simulink model "modelo_linear_v2"  (R2014b)
settings: Solver=ode45  StartTime=0.0  StopTime=T_sim  RelTol=1e-3
InitFcn:
  | main_v2
values from neighbouring files (symbols this model uses):
  Aw = A22(1:3,1:3)    [main_model2.m]    (also in main_modelo_linear_v1.m; main_modelo_linear_v2.m = zeros(6,6); main_modelo_nao_linear_v2.m)
  Bw = B22(1:3,1:3)    [main_model2.m]    (also in main_modelo_linear_v1.m; main_modelo_linear_v2.m = zeros(6,3); main_modelo_nao_linear_v2.m)
  Cw = eye(3)    [main_model2.m]    (also in main_modelo_linear_v1.m; main_modelo_linear_v2.m = eye(6); main_modelo_nao_linear_v2.m)
  Dw = zeros(3)    [main_model2.m]    (also in main_modelo_linear_v1.m; main_modelo_linear_v2.m = zeros(6,3); main_modelo_nao_linear_v2.m)
  g = 9.8    [main_model1.m]    (also in main_model2.m; main_modelo_linear_v1.m; main_modelo_linear_v2.m; main_modelo_nao_linear_v1.m)
  Kd_rot = 0.01    [main_model1.m]    (also in main_model2.m; main_modelo_linear_v1.m = 0; main_modelo_linear_v2.m = 0; main_modelo_nao_linear_v1.m)
  Kd_trans = 0.002    [main_model1.m]    (also in main_model2.m = -0.13723; main_modelo_linear_v1.m = 0; main_modelo_linear_v2.m = 0; main_modelo_nao_linear_v1.m)
  Ki_rot = 1.0    (= 1)    [main_model1.m]    (also in main_model2.m; main_modelo_linear_v1.m = 0.5; main_modelo_linear_v2.m = 0.5; main_modelo_nao_linear_v1.m)
  Ki_trans = 0.06    [main_model1.m]    (also in main_model2.m = 0.41774; main_modelo_linear_v1.m = 0; main_modelo_linear_v2.m = 1; main_modelo_nao_linear_v1.m)
  Kp_rot = 10    [main_model1.m]    (also in main_model2.m; main_modelo_linear_v1.m = 1; main_modelo_linear_v2.m = 1; main_modelo_nao_linear_v1.m)
  Kp_trans = 0.4    [main_model1.m]    (also in main_model2.m = 2.0968; main_modelo_linear_v1.m = 1; main_modelo_linear_v2.m = 2; main_modelo_nao_linear_v1.m)
  m = 1.0428    [main_model1.m]    (also in main_model2.m; main_modelo_linear_v1.m = 1; main_modelo_linear_v2.m = 1; main_modelo_nao_linear_v1.m)
  p0 = 0    [main_model2.m]    (also in main_modelo_linear_v1.m; main_modelo_linear_v2.m; main_modelo_nao_linear_v2.m; modelo_naolinear.m)
  phi0 = 0    [main_model1.m]    (also in main_model2.m; main_modelo_linear_v1.m; main_modelo_linear_v2.m; main_modelo_nao_linear_v1.m)
  psi0 = 0    [main_model1.m]    (also in main_model2.m; main_modelo_linear_v1.m; main_modelo_linear_v2.m; main_modelo_nao_linear_v1.m)
  q0 = 0    [main_model2.m]    (also in main_modelo_linear_v1.m; main_modelo_linear_v2.m; main_modelo_nao_linear_v2.m; modelo_naolinear.m)
  r0 = 0    [main_model2.m]    (also in main_modelo_linear_v1.m; main_modelo_linear_v2.m; main_modelo_nao_linear_v2.m; modelo_naolinear.m)
  theta0 = 0    [main_model1.m]    (also in main_model2.m; main_modelo_linear_v1.m; main_modelo_linear_v2.m; main_modelo_nao_linear_v1.m)
  vxd = 0    [main_model1.m]    (also in main_model2.m; main_modelo_linear_v1.m; main_modelo_linear_v2.m; main_modelo_nao_linear_v1.m)
  vyd = 0    [main_model1.m]    (also in main_model2.m; main_modelo_linear_v1.m; main_modelo_linear_v2.m; main_modelo_nao_linear_v1.m)
  x0 = 0    [main_model1.m]    (also in main_model2.m; main_modelo_linear_v1.m; main_modelo_linear_v2.m; main_modelo_nao_linear_v1.m)
  y0 = 0    [main_model1.m]    (also in main_model2.m; main_modelo_linear_v1.m; main_modelo_linear_v2.m; main_modelo_nao_linear_v1.m)
  z0 = 1    [main_model1.m]    (also in main_model2.m; main_modelo_linear_v1.m; main_modelo_linear_v2.m; main_modelo_nao_linear_v1.m)
undefined symbols (not defined in the file or in its folder): sigbuilder_block
libraries: simulink x6
settings Model: Creator=dferr  LastModifiedBy=dferr
settings DebuggingCC: SolverPrmCheckMsg=none

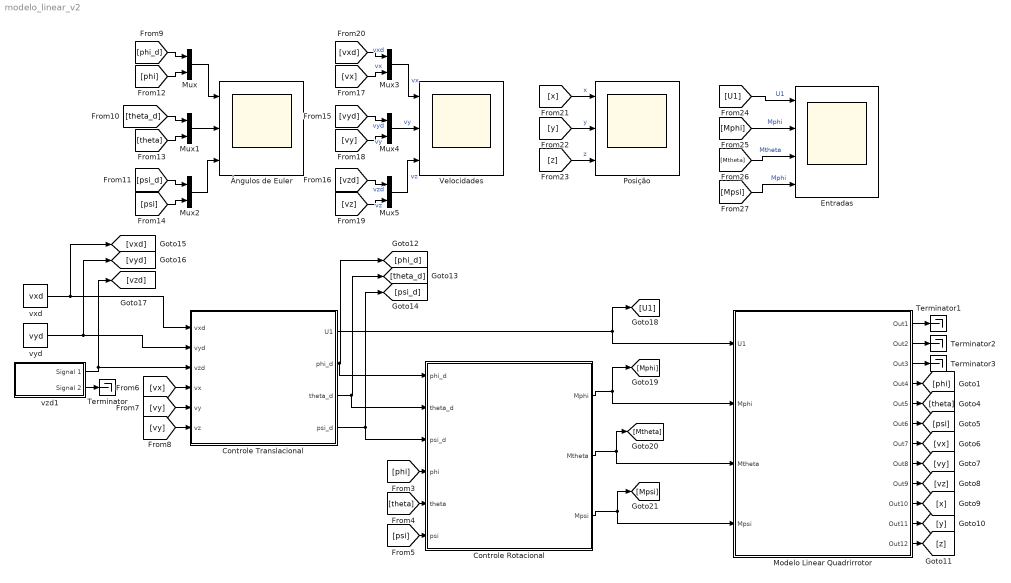
== system modelo_linear_v2 ==
  Controle Rotacional : Subsystem
      mask Display:
      | disp('Controle Rotacional')
      | port_label('input',1,'phi_d')
      | port_label('input',2,'theta_d')
      | port_label('input',3,'psi_d')
      | port_label('input',4,'phi')
      | port_label('input',5,'theta')
      | port_label('input',6,'psi')
      | port_label('output',1,'Mphi')
      | port_label('output',2,'Mtheta')
      | port_label('output',3,'Mpsi')
  Controle Translacional : Subsystem
      mask Display:
      | disp('Controle Translacional')
      | port_label('input',1,'vxd')
      | port_label('input',2,'vyd')
      | port_label('input',3,'vzd')
      | port_label('input',4,'vx')
      | port_label('input',5,'vy')
      | port_label('input',6,'vz')
      | port_label('output',1,'U1')
      | port_label('output',2,'phi_d')
      | port_label('output',3,'theta_d')
      | port_label('output',4,'psi_d')
  Entradas : Scope  NumInputPorts=4
      settings: YMin=-5~-5~-5~-5  YMax=5~5~5~5  SaveName=ScopeData3
  Modelo Linear Quadrirrotor : Subsystem
      mask Display:
      | disp('Modelo Linear Quadrirrotor')
      | port_label('input',1,'U1')
      | port_label('input',2,'Mphi')
      | port_label('input',3,'Mtheta')
      | port_label('input',4,'Mpsi')
      | port_label('output',1,'p')
      | port_label('output',2,'q')
      | port_label('output',3,'r')
      | port_label('output',4,'phi')
      | port_label('output',5,'theta')
      | port_label('output',6,'psi')
      | port_label('output',7,'vx')
      | port_label('output',8,'vy')
      | port_label('output',9,'vz')
      | port_label('output',10,'x')
      | port_label('output',11,'y')
      | port_label('output',12,'z')
  Mux{,1..5} (6 alike) : Mux  Inputs=2
  Posição : Scope  NumInputPorts=3
      settings: YMin=-5~-5~-5  YMax=5~5~5  SaveName=ScopeData2
  Terminator{,1..3} (4 alike) : Terminator
  Velocidades : Scope  NumInputPorts=3
      settings: ShowLegends=on  YMin=-5~-5~-5  YMax=5~5~5
  vxd : Constant  Value=vxd
  vyd : Constant  Value=vyd
  vzd1 : Subsystem  Tag=STV Subsys  LoadFcn=sigbuilder_block('load');  StartFcn=sigbuilder_block('start');  StopFcn=sigbuilder_block('stop');  ClipboardFcn=sigbuilder_block('clipboard');  mask(Sigbuilder block){}
      mask help: Simulink:masks:SigbuilderBlock_MD
      mask init:
      | if ~strcmp(get_param(bdroot(gcbh),'SimulationStatus'),'stopped') tuvar = sigbuilder_block('maskInit'); end
      settings: CopyFcn=sigbuilder_block('copy');  DeleteFcn=sigbuilder_block('delete');  ModelCloseFcn=sigbuilder_block('modelClose');  PreSaveFcn=sigbuilder_block('preSave');  PauseFcn=sigbuilder_block('pause');  ContinueFcn=sigbuilder_block('continue');  NameChangeFcn=sigbuilder_block('namechange');  OpenFcn=sigbuilder_block('open',[437.6 199.2 550.4 400 ]);  CloseFcn=sigbuilder_block('close');
      mask Display: plot(0, 0, 100, 100,[2, 2, 32, 32, 2], [68, 8, 8, 68, 68],[32, 2], [38, 38], [32, 19, 2],[53, 60, 44], [32, 17, 17, 2],[16, 16, 31, 31]);txt = getActiveGroup(gcbh);text(2, 100, txt,'verticalAlignment', 'top');
  Ângulos de Euler : Scope  NumInputPorts=3
      settings: YMin=-5~-5~-5  YMax=5~5~5
  wires:
  Controle Rotacional/1(Mphi) -> [Mphi], Modelo Linear Quadrirrotor/2(Mphi)
  Controle Rotacional/2(Mtheta) -> [Mtheta], Modelo Linear Quadrirrotor/3(Mtheta)
  Controle Rotacional/3(Mpsi) -> [Mpsi], Modelo Linear Quadrirrotor/4(Mpsi)
  Controle Translacional/4(psi_d) -> [psi_d], Controle Rotacional/3(psi_d)
  Controle Translacional/3(theta_d) -> Controle Rotacional/2(theta_d), [theta_d]
  Controle Translacional/2(phi_d) -> Controle Rotacional/1(phi_d), [phi_d]
  Controle Translacional/1(U1) -> [U1], Modelo Linear Quadrirrotor/1(U1)
  [vx] -> Controle Translacional/4(vx)
  [vy] -> Controle Translacional/5(vy)
  [vy] -> Controle Translacional/6(vz)
  vyd/1 -> [vyd], Controle Translacional/2(vyd)
  vxd/1 -> [vxd], Controle Translacional/1(vxd)
  [phi] -> Mux/2
  [phi_d] -> Mux/1
  [theta_d] -> Mux1/1
  [theta] -> Mux1/2
  [psi_d] -> Mux2/1
  [psi] -> Mux2/2
  Mux1/1 -> Ângulos de Euler/2
  Mux/1 -> Ângulos de Euler/1
  Mux2/1 -> Ângulos de Euler/3
  vzd1/2(Signal 2) -> Terminator/1
  [vx] -> Mux3/2  "vx"
  [vxd] -> Mux3/1  "vxd"
  [vyd] -> Mux4/1  "vyd"
  [vy] -> Mux4/2  "vy"
  [vzd] -> Mux5/1  "vzd"
  [vz] -> Mux5/2  "vz"
  Mux4/1 -> Velocidades/2  "vy"
  Mux3/1 -> Velocidades/1  "vx"
  Mux5/1 -> Velocidades/3  "vz"
  [x] -> Posição/1  "x"
  [y] -> Posição/2  "y"
  [z] -> Posição/3  "z"
  [U1] -> Entradas/1  "U1"
  [Mphi] -> Entradas/2  "Mphi"
  [Mtheta] -> Entradas/3  "Mtheta"
  [Mpsi] -> Entradas/4  "Mphi"
  vzd1/1(Signal 1) -> Controle Translacional/3(vzd), [vzd]
  Modelo Linear Quadrirrotor/1(Out1) -> Terminator1/1
  Modelo Linear Quadrirrotor/2(Out2) -> Terminator2/1
  Modelo Linear Quadrirrotor/3(Out3) -> Terminator3/1
  Modelo Linear Quadrirrotor/4(Out4) -> [phi]
  Modelo Linear Quadrirrotor/5(Out5) -> [theta]
  Modelo Linear Quadrirrotor/6(Out6) -> [psi]
  Modelo Linear Quadrirrotor/7(Out7) -> [vx]
  Modelo Linear Quadrirrotor/8(Out8) -> [vy]
  Modelo Linear Quadrirrotor/9(Out9) -> [vz]
  Modelo Linear Quadrirrotor/10(Out10) -> [x]
  Modelo Linear Quadrirrotor/11(Out11) -> [y]
  Modelo Linear Quadrirrotor/12(Out12) -> [z]
  [phi] -> Controle Rotacional/4(phi)
  [theta] -> Controle Rotacional/5(theta)
  [psi] -> Controle Rotacional/6(psi)

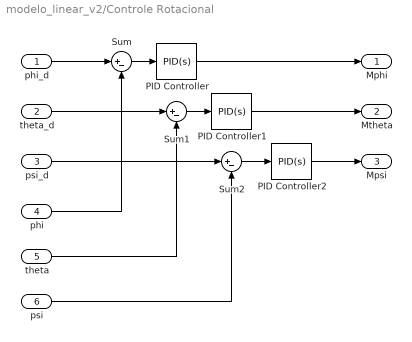
== system modelo_linear_v2/Controle Rotacional ==
  phi_d : Inport
  theta_d : Inport  Port=2
  psi_d : Inport  Port=3
  phi : Inport  Port=4
  theta : Inport  Port=5
  psi : Inport  Port=6
  PID Controller : simulink/Continuous/PID Controller  Controller=PID  TimeDomain=Continuous-time  SampleTime=-1  IntegratorMethod=Forward Euler  FilterMethod=Forward Euler  Form=Parallel  P=Kp_rot  I=Ki_rot  D=Kd_rot  N=100  InitialConditionSource=internal  InitialConditionForIntegrator=0  InitialConditionForFilter=0  ExternalReset=none  LimitOutput=off  UpperSaturationLimit=inf  LowerSaturationLimit=-inf  LinearizeAsGain=on  AntiWindupMode=none  Kb=1  TrackingMode=off  Kt=1  PParamMin=[]  PParamMax=[]  IParamMin=[]  IParamMax=[]  DParamMin=[]  DParamMax=[]  NParamMin=[]  NParamMax=[]  KbParamMin=[]  KbParamMax=[]  KtParamMin=[]  KtParamMax=[]  POutMin=[]  POutMax=[]  IOutMin=[]  IOutMax=[]  DOutMin=[]  DOutMax=[]  NOutMin=[]  NOutMax=[]  KbOutMin=[]  KbOutMax=[]  KtOutMin=[]  KtOutMax=[]  IntegratorOutMin=[]  IntegratorOutMax=[]  FilterOutMin=[]  FilterOutMax=[]  SumOutMin=[]  SumOutMax=[]  SumI1OutMin=[]  SumI1OutMax=[]  SumI2OutMin=[]  SumI2OutMax=[]  SumI3OutMin=[]  SumI3OutMax=[]  SumDOutMin=[]  SumDOutMax=[]  SaturationOutMin=[]  SaturationOutMax=[]  IntegratorContinuousStateAttributes=''  IntegratorStateMustResolveToSignalObject=off  IntegratorRTWStateStorageClass=Auto  FilterContinuousStateAttributes=''  FilterStateMustResolveToSignalObject=off  FilterRTWStateStorageClass=Auto  DifferentiatorICPrevScaledInput=0  DifferentiatorOutMin=[]  DifferentiatorOutMax=[]  UseFilter=on
  PID Controller1 : simulink/Continuous/PID Controller  Controller=PID  TimeDomain=Continuous-time  SampleTime=-1  IntegratorMethod=Forward Euler  FilterMethod=Forward Euler  Form=Parallel  P=Kp_rot  I=Ki_rot  D=Kd_rot  N=100  InitialConditionSource=internal  InitialConditionForIntegrator=0  InitialConditionForFilter=0  ExternalReset=none  LimitOutput=off  UpperSaturationLimit=inf  LowerSaturationLimit=-inf  LinearizeAsGain=on  AntiWindupMode=none  Kb=1  TrackingMode=off  Kt=1  PParamMin=[]  PParamMax=[]  IParamMin=[]  IParamMax=[]  DParamMin=[]  DParamMax=[]  NParamMin=[]  NParamMax=[]  KbParamMin=[]  KbParamMax=[]  KtParamMin=[]  KtParamMax=[]  POutMin=[]  POutMax=[]  IOutMin=[]  IOutMax=[]  DOutMin=[]  DOutMax=[]  NOutMin=[]  NOutMax=[]  KbOutMin=[]  KbOutMax=[]  KtOutMin=[]  KtOutMax=[]  IntegratorOutMin=[]  IntegratorOutMax=[]  FilterOutMin=[]  FilterOutMax=[]  SumOutMin=[]  SumOutMax=[]  SumI1OutMin=[]  SumI1OutMax=[]  SumI2OutMin=[]  SumI2OutMax=[]  SumI3OutMin=[]  SumI3OutMax=[]  SumDOutMin=[]  SumDOutMax=[]  SaturationOutMin=[]  SaturationOutMax=[]  IntegratorContinuousStateAttributes=''  IntegratorStateMustResolveToSignalObject=off  IntegratorRTWStateStorageClass=Auto  FilterContinuousStateAttributes=''  FilterStateMustResolveToSignalObject=off  FilterRTWStateStorageClass=Auto  DifferentiatorICPrevScaledInput=0  DifferentiatorOutMin=[]  DifferentiatorOutMax=[]  UseFilter=on
  PID Controller2 : simulink/Continuous/PID Controller  Controller=PID  TimeDomain=Continuous-time  SampleTime=-1  IntegratorMethod=Forward Euler  FilterMethod=Forward Euler  Form=Parallel  P=Kp_rot  I=Ki_rot  D=Kd_rot  N=100  InitialConditionSource=internal  InitialConditionForIntegrator=0  InitialConditionForFilter=0  ExternalReset=none  LimitOutput=off  UpperSaturationLimit=inf  LowerSaturationLimit=-inf  LinearizeAsGain=on  AntiWindupMode=none  Kb=1  TrackingMode=off  Kt=1  PParamMin=[]  PParamMax=[]  IParamMin=[]  IParamMax=[]  DParamMin=[]  DParamMax=[]  NParamMin=[]  NParamMax=[]  KbParamMin=[]  KbParamMax=[]  KtParamMin=[]  KtParamMax=[]  POutMin=[]  POutMax=[]  IOutMin=[]  IOutMax=[]  DOutMin=[]  DOutMax=[]  NOutMin=[]  NOutMax=[]  KbOutMin=[]  KbOutMax=[]  KtOutMin=[]  KtOutMax=[]  IntegratorOutMin=[]  IntegratorOutMax=[]  FilterOutMin=[]  FilterOutMax=[]  SumOutMin=[]  SumOutMax=[]  SumI1OutMin=[]  SumI1OutMax=[]  SumI2OutMin=[]  SumI2OutMax=[]  SumI3OutMin=[]  SumI3OutMax=[]  SumDOutMin=[]  SumDOutMax=[]  SaturationOutMin=[]  SaturationOutMax=[]  IntegratorContinuousStateAttributes=''  IntegratorStateMustResolveToSignalObject=off  IntegratorRTWStateStorageClass=Auto  FilterContinuousStateAttributes=''  FilterStateMustResolveToSignalObject=off  FilterRTWStateStorageClass=Auto  DifferentiatorICPrevScaledInput=0  DifferentiatorOutMin=[]  DifferentiatorOutMax=[]  UseFilter=on
  Sum : Sum  Inputs=|+-
  Sum1 : Sum  Inputs=|+-
  Sum2 : Sum  Inputs=|+-
  Mphi : Outport
  Mtheta : Outport  Port=2
  Mpsi : Outport  Port=3
  wires:
  PID Controller1/1 -> Mtheta/1
  PID Controller/1 -> Mphi/1
  PID Controller2/1 -> Mpsi/1
  Sum/1 -> PID Controller/1
  Sum1/1 -> PID Controller1/1
  Sum2/1 -> PID Controller2/1
  phi_d/1 -> Sum/1
  theta_d/1 -> Sum1/1
  psi_d/1 -> Sum2/1
  phi/1 -> Sum/2
  theta/1 -> Sum1/2
  psi/1 -> Sum2/2

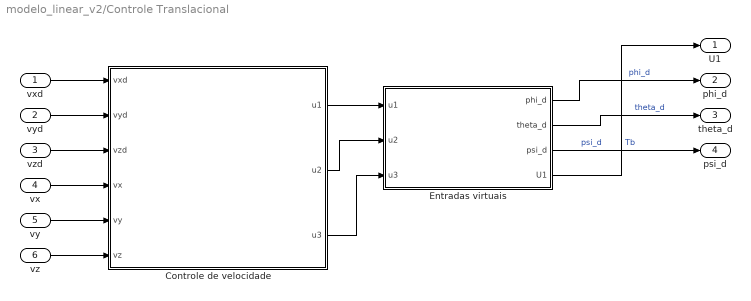
== system modelo_linear_v2/Controle Translacional ==
  vxd : Inport
  vyd : Inport  Port=2
  vzd : Inport  Port=3
  vx : Inport  Port=4
  vy : Inport  Port=5
  vz : Inport  Port=6
  Controle de velocidade : Subsystem
      mask Display:
      | disp('Controle de Velocidade PID')
      | port_label('input',1,'vxd')
      | port_label('input',2,'vyd')
      | port_label('input',3,'vzd')
      | port_label('input',4,'vx')
      | port_label('input',5,'vy')
      | port_label('input',6,'vz')
      | 
      | port_label('output',1,'u1')
      | port_label('output',2,'u2')
      | port_label('output',3,'u3')
  Entradas virtuais : Subsystem
      mask Display:
      | disp('(u1,u2,u3)->(eta_d,U1)')
      | port_label('input',1,'u1')
      | port_label('input',2,'u2')
      | port_label('input',3,'u3')
      | port_label('output',1,'phi_d')
      | port_label('output',2,'theta_d')
      | port_label('output',3,'psi_d')
      | port_label('output',4,'U1')
  U1 : Outport
  phi_d : Outport  Port=2
  theta_d : Outport  Port=3
  psi_d : Outport  Port=4
  wires:
  Controle de velocidade/2(u2) -> Entradas virtuais/2(u2)
  Entradas virtuais/1(phi_d) -> phi_d/1  "phi_d"
  Entradas virtuais/2(theta_d) -> theta_d/1  "theta_d"
  Entradas virtuais/3(psi_d) -> psi_d/1  "psi_d"
  Controle de velocidade/1(u1) -> Entradas virtuais/1(u1)
  vz/1 -> Controle de velocidade/6(vz)
  vy/1 -> Controle de velocidade/5("vy ")
  Controle de velocidade/3(u3) -> Entradas virtuais/3(u3)
  vx/1 -> Controle de velocidade/4(vx)
  Entradas virtuais/4(U1) -> U1/1  "Tb"
  vyd/1 -> Controle de velocidade/2(vyd)
  vzd/1 -> Controle de velocidade/3(vzd)
  vxd/1 -> Controle de velocidade/1(vxd)

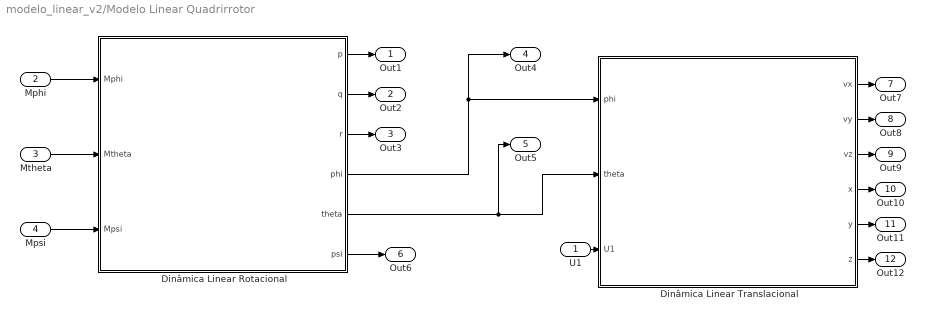
== system modelo_linear_v2/Modelo Linear Quadrirrotor ==
  U1 : Inport
  Mphi : Inport  Port=2
  Mtheta : Inport  Port=3
  Mpsi : Inport  Port=4
  Dinâmica Linear Rotacional : Subsystem
      mask Display:
      | disp('Dinâmica Linear Rotacional')
      | port_label('input',1,'Mphi')
      | port_label('input',2,'Mtheta')
      | port_label('input',3,'Mpsi')
      | port_label('output',1,'p')
      | port_label('output',2,'q')
      | port_label('output',3,'r')
      | port_label('output',4,'phi')
      | port_label('output',5,'theta')
      | port_label('output',6,'psi')
  Dinâmica Linear Translacional : Subsystem
      mask Display:
      | disp('Dinâmica Linear Translacional')
      | port_label('input',1,'phi')
      | port_label('input',2,'theta')
      | port_label('input',3,'U1')
      | port_label('output',1,'vx')
      | port_label('output',2,'vy')
      | port_label('output',3,'vz')
      | port_label('output',4,'x')
      | port_label('output',5,'y')
      | port_label('output',6,'z')
  Out1 : Outport
  Out2 : Outport  Port=2
  Out3 : Outport  Port=3
  Out4 : Outport  Port=4
  Out5 : Outport  Port=5
  Out6 : Outport  Port=6
  Out7 : Outport  Port=7
  Out8 : Outport  Port=8
  Out9 : Outport  Port=9
  Out10 : Outport  Port=10
  Out11 : Outport  Port=11
  Out12 : Outport  Port=12
  wires:
  Mphi/1 -> Dinâmica Linear Rotacional/1(Mphi)
  Mtheta/1 -> Dinâmica Linear Rotacional/2(Mtheta)
  Mpsi/1 -> Dinâmica Linear Rotacional/3(Mpsi)
  U1/1 -> Dinâmica Linear Translacional/3(U1)
  Dinâmica Linear Rotacional/4(phi) -> Out4/1, Dinâmica Linear Translacional/1(phi)
  Dinâmica Linear Rotacional/5(theta) -> Out5/1, Dinâmica Linear Translacional/2(theta)
  Dinâmica Linear Rotacional/1(p) -> Out1/1
  Dinâmica Linear Rotacional/2(q) -> Out2/1
  Dinâmica Linear Rotacional/3(r) -> Out3/1
  Dinâmica Linear Rotacional/6(psi) -> Out6/1
  Dinâmica Linear Translacional/1(vx) -> Out7/1
  Dinâmica Linear Translacional/2(vy) -> Out8/1
  Dinâmica Linear Translacional/3(vz) -> Out9/1
  Dinâmica Linear Translacional/4(x) -> Out10/1
  Dinâmica Linear Translacional/5(y) -> Out11/1
  Dinâmica Linear Translacional/6(z) -> Out12/1

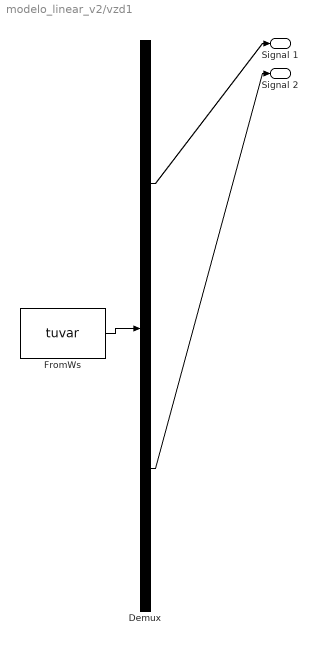
== system modelo_linear_v2/vzd1 ==
  Demux : Demux  Tag=STV Demux  Outputs=2
  FromWs : FromWorkspace  Tag=STV FromWs  VariableName=tuvar  SampleTime=0
      SigBuilderData=|
      | common.afterFinalStr = 'Extrapolate'
      | common.sampleTime = 0
      | dataSet.timeRange = [0 20]
      | dataSet.name = 'Group 1'
      | sbobj.Groups.Name = 'Group 1'
      | sbobj.Groups.Signals(1).Name = 'Signal 1'
      | sbobj.Groups.Signals(1).XData = [0 2.05 4.75 8 14 18 20]
      | sbobj.Groups.Signals(1).YData = [0.005 0.215 0.215 -0.12 -0.12 0 0]
      | sbobj.Groups.Signals(2).Name = 'Signal 2'
      | sbobj.Groups.Signals(2).XData = [0 5 5 20]
      | sbobj.Groups.Signals(2).YData = [0 0 1 1]
      | sbobj.Groups.TimeRange = [0 20]
  Signal 1 : Outport  Tag=STV Outport
  Signal 2 : Outport  Tag=STV Outport  Port=2
  wires:
  FromWs/1 -> Demux/1
  Demux/1 -> Signal 1/1
  Demux/2 -> Signal 2/1

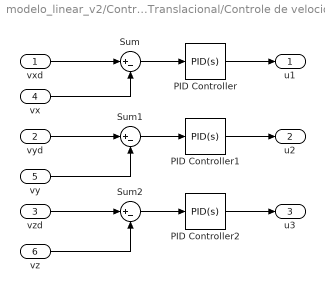
== system modelo_linear_v2/Controle Translacional/Controle de velocidade ==
  vxd : Inport
  vyd : Inport  Port=2
  vzd : Inport  Port=3
  vx : Inport  Port=4
  "vy " : Inport  Port=5
  vz : Inport  Port=6
  PID Controller : simulink/Continuous/PID Controller  Controller=PID  TimeDomain=Continuous-time  SampleTime=-1  IntegratorMethod=Forward Euler  FilterMethod=Forward Euler  Form=Parallel  P=Kp_trans  I=Ki_trans  D=Kd_trans  N=100  InitialConditionSource=internal  InitialConditionForIntegrator=0  InitialConditionForFilter=0  ExternalReset=none  LimitOutput=off  UpperSaturationLimit=inf  LowerSaturationLimit=-inf  LinearizeAsGain=on  AntiWindupMode=none  Kb=1  TrackingMode=off  Kt=1  RndMeth=Nearest  PParamMin=[]  PParamMax=[]  IParamMin=[]  IParamMax=[]  DParamMin=[]  DParamMax=[]  NParamMin=[]  NParamMax=[]  KbParamMin=[]  KbParamMax=[]  KtParamMin=[]  KtParamMax=[]  POutMin=[]  POutMax=[]  IOutMin=[]  IOutMax=[]  DOutMin=[]  DOutMax=[]  NOutMin=[]  NOutMax=[]  KbOutMin=[]  KbOutMax=[]  KtOutMin=[]  KtOutMax=[]  IntegratorOutMin=[]  IntegratorOutMax=[]  FilterOutMin=[]  FilterOutMax=[]  SumOutMin=[]  SumOutMax=[]  SumI1OutMin=[]  SumI1OutMax=[]  SumI2OutMin=[]  SumI2OutMax=[]  SumI3OutMin=[]  SumI3OutMax=[]  SumDOutMin=[]  SumDOutMax=[]  SaturationOutMin=[]  SaturationOutMax=[]  IntegratorContinuousStateAttributes=''  IntegratorStateMustResolveToSignalObject=off  IntegratorRTWStateStorageClass=Auto  FilterContinuousStateAttributes=''  FilterStateMustResolveToSignalObject=off  FilterRTWStateStorageClass=Auto  DifferentiatorICPrevScaledInput=0  DifferentiatorOutMin=[]  DifferentiatorOutMax=[]  UseFilter=on
      settings: LockScale=on
  PID Controller1 : simulink/Continuous/PID Controller  Controller=PID  TimeDomain=Continuous-time  SampleTime=-1  IntegratorMethod=Forward Euler  FilterMethod=Forward Euler  Form=Parallel  P=Kp_trans  I=Ki_trans  D=Kd_trans  N=100  InitialConditionSource=internal  InitialConditionForIntegrator=0  InitialConditionForFilter=0  ExternalReset=none  LimitOutput=off  UpperSaturationLimit=inf  LowerSaturationLimit=-inf  LinearizeAsGain=on  AntiWindupMode=none  Kb=1  TrackingMode=off  Kt=1  RndMeth=Nearest  PParamMin=[]  PParamMax=[]  IParamMin=[]  IParamMax=[]  DParamMin=[]  DParamMax=[]  NParamMin=[]  NParamMax=[]  KbParamMin=[]  KbParamMax=[]  KtParamMin=[]  KtParamMax=[]  POutMin=[]  POutMax=[]  IOutMin=[]  IOutMax=[]  DOutMin=[]  DOutMax=[]  NOutMin=[]  NOutMax=[]  KbOutMin=[]  KbOutMax=[]  KtOutMin=[]  KtOutMax=[]  IntegratorOutMin=[]  IntegratorOutMax=[]  FilterOutMin=[]  FilterOutMax=[]  SumOutMin=[]  SumOutMax=[]  SumI1OutMin=[]  SumI1OutMax=[]  SumI2OutMin=[]  SumI2OutMax=[]  SumI3OutMin=[]  SumI3OutMax=[]  SumDOutMin=[]  SumDOutMax=[]  SaturationOutMin=[]  SaturationOutMax=[]  IntegratorContinuousStateAttributes=''  IntegratorStateMustResolveToSignalObject=off  IntegratorRTWStateStorageClass=Auto  FilterContinuousStateAttributes=''  FilterStateMustResolveToSignalObject=off  FilterRTWStateStorageClass=Auto  DifferentiatorICPrevScaledInput=0  DifferentiatorOutMin=[]  DifferentiatorOutMax=[]  UseFilter=on
      settings: LockScale=on
  PID Controller2 : simulink/Continuous/PID Controller  Controller=PID  TimeDomain=Continuous-time  SampleTime=-1  IntegratorMethod=Forward Euler  FilterMethod=Forward Euler  Form=Parallel  P=Kp_trans  I=Ki_trans  D=Kd_trans  N=100  InitialConditionSource=internal  InitialConditionForIntegrator=0  InitialConditionForFilter=0  ExternalReset=none  LimitOutput=off  UpperSaturationLimit=inf  LowerSaturationLimit=-inf  LinearizeAsGain=on  AntiWindupMode=none  Kb=1  TrackingMode=off  Kt=1  RndMeth=Nearest  PParamMin=[]  PParamMax=[]  IParamMin=[]  IParamMax=[]  DParamMin=[]  DParamMax=[]  NParamMin=[]  NParamMax=[]  KbParamMin=[]  KbParamMax=[]  KtParamMin=[]  KtParamMax=[]  POutMin=[]  POutMax=[]  IOutMin=[]  IOutMax=[]  DOutMin=[]  DOutMax=[]  NOutMin=[]  NOutMax=[]  KbOutMin=[]  KbOutMax=[]  KtOutMin=[]  KtOutMax=[]  IntegratorOutMin=[]  IntegratorOutMax=[]  FilterOutMin=[]  FilterOutMax=[]  SumOutMin=[]  SumOutMax=[]  SumI1OutMin=[]  SumI1OutMax=[]  SumI2OutMin=[]  SumI2OutMax=[]  SumI3OutMin=[]  SumI3OutMax=[]  SumDOutMin=[]  SumDOutMax=[]  SaturationOutMin=[]  SaturationOutMax=[]  IntegratorContinuousStateAttributes=''  IntegratorStateMustResolveToSignalObject=off  IntegratorRTWStateStorageClass=Auto  FilterContinuousStateAttributes=''  FilterStateMustResolveToSignalObject=off  FilterRTWStateStorageClass=Auto  DifferentiatorICPrevScaledInput=0  DifferentiatorOutMin=[]  DifferentiatorOutMax=[]  UseFilter=on
      settings: LockScale=on
  Sum : Sum  Inputs=|+-
  Sum1 : Sum  Inputs=|+-
  Sum2 : Sum  Inputs=|+-
  u1 : Outport
  u2 : Outport  Port=2
  u3 : Outport  Port=3
  wires:
  vxd/1 -> Sum/1
  vz/1 -> Sum2/2
  vyd/1 -> Sum1/1
  vzd/1 -> Sum2/1
  vx/1 -> Sum/2
  "vy "/1 -> Sum1/2
  Sum/1 -> PID Controller/1
  PID Controller/1 -> u1/1
  Sum2/1 -> PID Controller2/1
  PID Controller2/1 -> u3/1
  PID Controller1/1 -> u2/1
  Sum1/1 -> PID Controller1/1

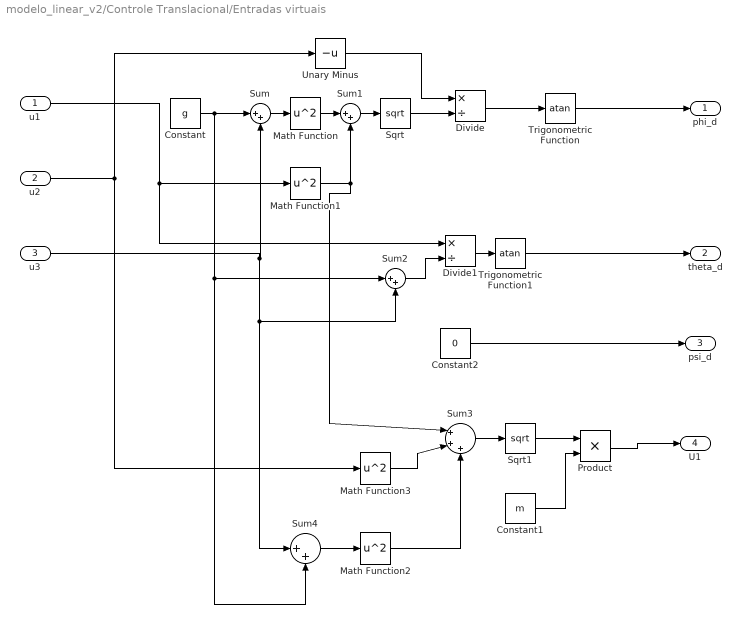
== system modelo_linear_v2/Controle Translacional/Entradas virtuais ==
  u1 : Inport
  u2 : Inport  Port=2
  u3 : Inport  Port=3
  Constant : Constant  Value=g
  Constant1 : Constant  Value=m
  Constant2 : Constant  Value=0
  Divide : Product  Inputs=*/
  Divide1 : Product  Inputs=*/
  Math Function{,1..3} (4 alike) : Math  Operator=square  SaturateOnIntegerOverflow=on
  Product : Product
  Sqrt : Sqrt  SaturateOnIntegerOverflow=on
  Sqrt1 : Sqrt  SaturateOnIntegerOverflow=on
  Sum{,1..2,4} (4 alike) : Sum  Inputs=|++
  Sum3 : Sum  Inputs=|+++
  Trigonometric Function : Trigonometry  Operator=atan
  Trigonometric Function1 : Trigonometry  Operator=atan
  Unary Minus : UnaryMinus
  phi_d : Outport
  theta_d : Outport  Port=2
  psi_d : Outport  Port=3
  U1 : Outport  Port=4
  wires:
  Divide/1 -> Trigonometric Function/1
  Sqrt/1 -> Divide/2
  Trigonometric Function1/1 -> theta_d/1
  Sum1/1 -> Sqrt/1
  Divide1/1 -> Trigonometric Function1/1
  Sum/1 -> Math Function/1
  u1/1 -> Divide1/1, Math Function1/1
  Trigonometric Function/1 -> phi_d/1
  Sum2/1 -> Divide1/2
  Constant1/1 -> Product/2
  Math Function3/1 -> Sum3/2
  u2/1 -> Math Function3/1, Unary Minus/1
  Constant2/1 -> psi_d/1
  Sqrt1/1 -> Product/1
  Sum3/1 -> Sqrt1/1
  Math Function2/1 -> Sum3/3
  u3/1 -> Sum4/1, Sum2/2, Sum/2
  Constant/1 -> Sum4/2, Sum2/1, Sum/1
  Math Function/1 -> Sum1/1
  Product/1 -> U1/1
  Math Function1/1 -> Sum3/1, Sum1/2
  Sum4/1 -> Math Function2/1
  Unary Minus/1 -> Divide/1

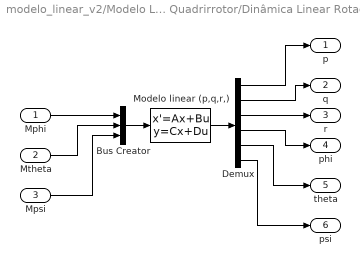
== system modelo_linear_v2/Modelo Linear Quadrirrotor/Dinâmica Linear Rotacional ==
  Mphi : Inport
  Mtheta : Inport  Port=2
  Mpsi : Inport  Port=3
  Bus Creator : BusCreator  Inputs=3
  Demux : Demux  Outputs=6
  "Modelo linear (p,q,r,) " : StateSpace  A=Aw  B=Bw  C=Cw  D=Dw  X0=[p0,q0,r0,phi0,theta0,psi0]
  p : Outport
  q : Outport  Port=2
  r : Outport  Port=3
  phi : Outport  Port=4
  theta : Outport  Port=5
  psi : Outport  Port=6
  wires:
  Bus Creator/1 -> "Modelo linear (p,q,r,) "/1
  Mpsi/1 -> Bus Creator/3
  Mphi/1 -> Bus Creator/1
  Mtheta/1 -> Bus Creator/2
  "Modelo linear (p,q,r,) "/1 -> Demux/1
  Demux/1 -> p/1
  Demux/2 -> q/1
  Demux/3 -> r/1
  Demux/4 -> phi/1
  Demux/5 -> theta/1
  Demux/6 -> psi/1

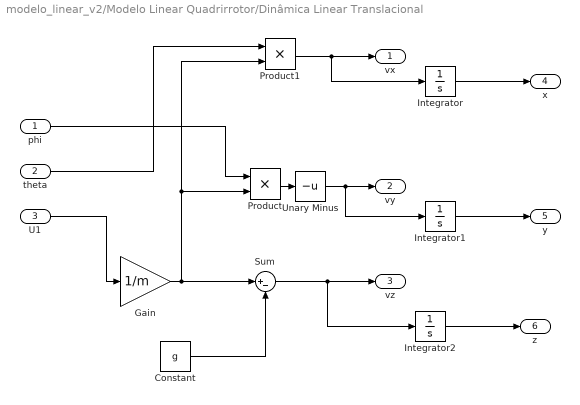
== system modelo_linear_v2/Modelo Linear Quadrirrotor/Dinâmica Linear Translacional ==
  phi : Inport
  theta : Inport  Port=2
  U1 : Inport  Port=3
  Constant : Constant  Value=g
  Gain : Gain  Gain=1/m
  Integrator : Integrator  InitialCondition=x0
  Integrator1 : Integrator  InitialCondition=y0
  Integrator2 : Integrator  InitialCondition=z0
  Product : Product
  Product1 : Product
  Sum : Sum  Inputs=|+-
  Unary Minus : UnaryMinus
  vx : Outport
  vy : Outport  Port=2
  vz : Outport  Port=3
  x : Outport  Port=4
  y : Outport  Port=5
  z : Outport  Port=6
  wires:
  Integrator1/1 -> y/1
  U1/1 -> Gain/1
  Integrator/1 -> x/1
  Integrator2/1 -> z/1
  Product1/1 -> vx/1, Integrator/1
  Gain/1 -> Sum/1, Product/2, Product1/2
  phi/1 -> Product/1
  theta/1 -> Product1/1
  Product/1 -> Unary Minus/1
  Unary Minus/1 -> Integrator1/1, vy/1
  Sum/1 -> Integrator2/1, vz/1
  Constant/1 -> Sum/2
